simulink model "part_f_nonlinear"  (R2024b)
settings: Solver=VariableStepAuto  StartTime=0.0  StopTime=50  RelTol=1e-3
values from neighbouring files (symbols this model uses):
  g = sym("g")    [part_E.m]    (also in part_F.m = 9.8; part_G.m = 9.8; part_b.m; part_c.m)
  l1 = sym("l1")    [part_E.m]    (also in part_F.m = 20; part_G.m = 20; part_b.m; part_c.m)
  l2 = sym("l2")    [part_E.m]    (also in part_F.m = 10; part_G.m = 10; part_b.m; part_c.m)
  M = sym("M")    [part_E.m]    (also in part_F.m = 1000; part_G.m = 1000; part_b.m; part_c.m)
  m1 = sym("m1")    [part_E.m]    (also in part_F.m = 100; part_G.m = 100; part_b.m; part_c.m)
  m2 = sym("m2")    [part_E.m]    (also in part_F.m = 100; part_G.m = 100; part_b.m; part_c.m)
undefined symbols (not defined in the file or in its folder): L1, L3, L4
settings Model: Creator=timsweeney  LastModifiedBy=grays

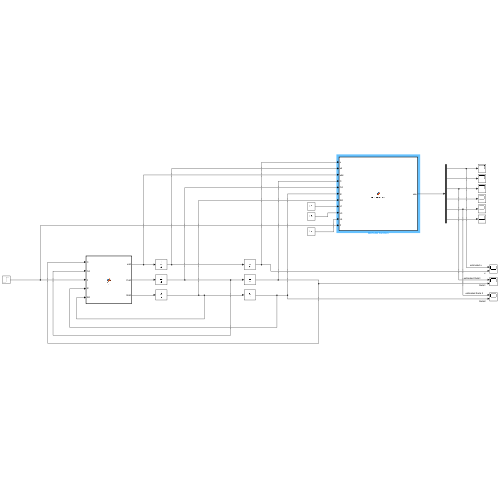
[thumbnail: Simulink's stored preview of the top-level diagram]
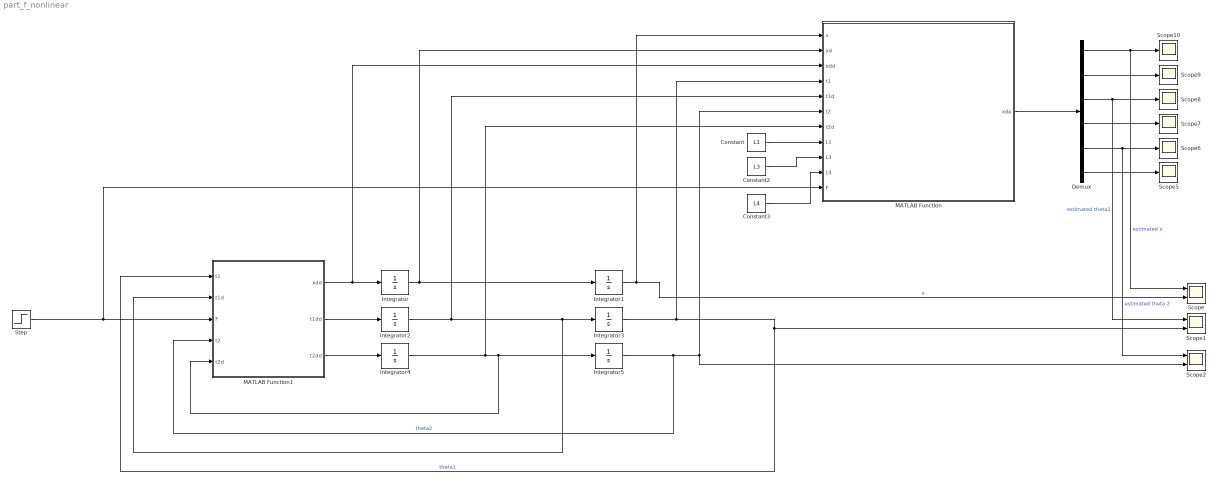
== system part_f_nonlinear ==
  Constant : Constant  Value=L1
  Constant2 : Constant  Value=L3
  Constant3 : Constant  Value=L4
  Demux : Demux  Outputs=6
  Integrator{,1..5} (6 alike) : Integrator
  MATLAB Function : MATLAB Function  TreatAsAtomicUnit=on
  MATLAB Function1 : MATLAB Function  TreatAsAtomicUnit=on
  Scope : Scope  NumInputPorts=2
  Scope1 : Scope  NumInputPorts=2
  Scope{5..10} (6 alike) : Scope
  Scope2 : Scope  NumInputPorts=2
  Step : Step  SampleTime=0
  wires:
  MATLAB Function1/1(xdd) -> MATLAB Function/3(xdd), Integrator/1
  MATLAB Function1/2(t1dd) -> Integrator2/1
  Integrator/1 -> MATLAB Function/2(xd), Integrator1/1
  Integrator2/1 -> MATLAB Function/5(t1d), Integrator3/1, MATLAB Function1/2(t1d)
  Integrator4/1 -> MATLAB Function/7(t2d), Integrator5/1, MATLAB Function1/5(t2d)
  Integrator1/1 -> MATLAB Function/1(x), Scope/2  "x"
  Integrator3/1 -> MATLAB Function/4(t1), MATLAB Function1/1(t1), Scope1/2  "theta1"
  Integrator5/1 -> Scope2/2, MATLAB Function/6(t2), MATLAB Function1/4(t2)  "theta2"
  MATLAB Function1/3(t2dd) -> Integrator4/1
  Constant/1 -> MATLAB Function/8(L1)
  MATLAB Function/1(xde) -> Demux/1
  Demux/1 -> Scope/1, Scope10/1  "estimated x"
  Demux/4 -> Scope7/1
  Demux/3 -> Scope1/1, Scope8/1  "estimated theta1"
  Demux/2 -> Scope9/1
  Demux/5 -> Scope2/1, Scope6/1  "estimated theta 2"
  Demux/6 -> Scope5/1
  Constant2/1 -> MATLAB Function/9(L3)
  Constant3/1 -> MATLAB Function/10(L4)
  Step/1 -> MATLAB Function/11(F), MATLAB Function1/3(F)

== matlab function part_f_nonlinear/MATLAB Function1 ==
  data: t1 input; t1d input; F input; t2 input; t2d input; xdd output; t1dd output; m1 parameter; m2 parameter; l1 parameter; l2 parameter; M parameter; g parameter; t2dd output
function [xdd, t1dd, t2dd] = fcn( t1, t1d, F, t2, t2d, m1, m2, l1, l2, M, g)

xdd = (F - m1*l1*sin(t1)*t1d^2 - m2*l2*sin(t2)*t2d^2 - m1*g*cos(t1)*sin(t1) - m2*g*cos(t2)*sin(t2)) ...
       / ...
      (M + m1*sin(t1)^2 + m2*sin(t2)^2);
t1dd = (1/l1) * (cos(t1)*xdd - g*sin(t1));
t2dd = (1/l2) * (cos(t2)*xdd - g*sin(t2));

% t2dd = 0;

== matlab function part_f_nonlinear/MATLAB Function ==
  data: x input; xd input; xdd input; t1 input; t1d input; t2 input; t2d input; xde output; L1 input; L3 input; L4 input; F input
function xde  = observerfcn( x, xd, xdd, t1, t1d, t2, t2d, L1, L3, L4, F)

g = 9.81;
m1 = 100;
m2 = 100;
M = 1000;
l1 = 20;
l2 = 10;
xde = zeros(6,1);

current_y = [x; xd; t1; t1d; t2; t2d];

% Uncomment lines of code based on which output vector you are observing

y1 = [x];
c1 = [1, 0, 0, 0, 0, 0];
est = L1 * (y1 - (c1*current_y));

%y3 = [x; t2];
%c3 = [1, 0, 0, 0, 0, 0; 0, 0, 0, 0, 1, 0];
%est = L3 * (y3 - (c3*current_y));

%y4 = [x; t1; t2];
%c4 = [1, 0, 0, 0, 0, 0; 0, 0, 1, 0, 0, 0; 0, 0, 0, 0, 1, 0];
%est = L4 * (y4 - (c4*current_y));

xde(1) = xd + est(1);
xde(2) = ((F - m1*l1*sin(t1)*t1d^2 - m2*l2*sin(t2)*t2d^2 - m1*g*cos(t1)*sin(t1) - m2*g*cos(t2)*sin(t2)) ...
       / ...
      (M + m1*sin(t1)^2 + m2*sin(t2)^2)) + est(2);
xde(3) = t1d + est(3);
xde(4) = (1/l1) * (cos(t1)*xdd - g*sin(t1)) + est(4);
xde(5) = t2d + est(5);
xde(6) = (1/l2) * (cos(t2)*xdd - g*sin(t2)) + est(6);
